simulink model "Main_system"  (R2016a)
settings: Solver=VariableStepAuto  StartTime=0.0  StopTime=10.0  RelTol=1e-3
libraries: simulink x1
settings Model: Creator=hi  LastModifiedBy=hi

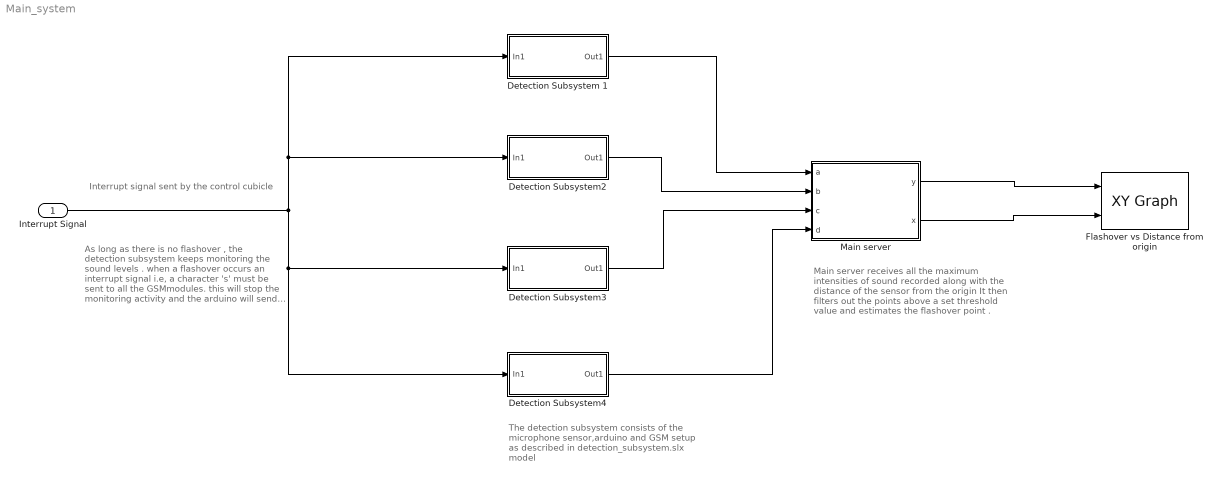
== system Main_system ==
  note: The detection subsystem consists
      | of the microphone sensor,arduino and
      | GSM setup as described in
      | detection_subsystem.slx model
  note: Main server receives all the maximum
      | intensities of sound recorded along with
      | the distance of the sensor from the origin
      |
      | It then filters out the points above a set
      | threshold value and estimates  the
      | flashover point .
  note: As long as there is no flashover , the
      | detection subsystem keeps monitoring
      | the sound levels .
      |
      | when a flashover occurs an interrupt
      | signal i.e, a character 's' must be sent to
      | all the GSMmodules.
      |
      | this will stop the monitoring activity
      | and the arduino will send the latest
      | sampled data to the web server
      | which will calculate the flashover
      | point.
  note: Interrupt signal sent by the control cubicle
  "Interrupt Signal " : Inport
  Detection Subsystem 1 : Subsystem
  Detection Subsystem2 : Subsystem
  Detection Subsystem3 : Subsystem
  Detection Subsystem4 : Subsystem
  Flashover vs Distance from origin : simulink/Sinks/XY Graph  xmin=-1  xmax=1  ymin=-1  ymax=1  st=-1
  Main server : MATLAB Function  TreatAsAtomicUnit=on
  wires:
  "Interrupt Signal "/1 -> Detection Subsystem4/1(In1), Detection Subsystem3/1(In1), Detection Subsystem 1/1(In1), Detection Subsystem2/1(In1)
  Detection Subsystem 1/1(Out1) -> Main server/1(a)
  Detection Subsystem2/1(Out1) -> Main server/2(b)
  Detection Subsystem3/1(Out1) -> Main server/3(c)
  Detection Subsystem4/1(Out1) -> Main server/4(d)
  Main server/1(y) -> Flashover vs Distance from origin/1
  Main server/2(x) -> Flashover vs Distance from origin/2

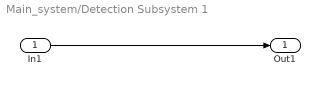
== system Main_system/Detection Subsystem 1 ==
  In1 : Inport
  Out1 : Outport
  wires:
  In1/1 -> Out1/1

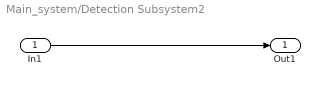
== system Main_system/Detection Subsystem2 ==
  In1 : Inport
  Out1 : Outport
  wires:
  In1/1 -> Out1/1

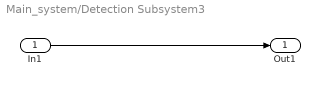
== system Main_system/Detection Subsystem3 ==
  In1 : Inport
  Out1 : Outport
  wires:
  In1/1 -> Out1/1

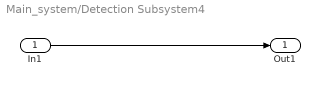
== system Main_system/Detection Subsystem4 ==
  In1 : Inport
  Out1 : Outport
  wires:
  In1/1 -> Out1/1

== matlab function Main_system/Main server ==
  data: a input; y output; b input; c input; d input; x output
function [y,x] = fcn(a,b,c,d)
%#codegen

y = u;
